simulink model "BATTERY_closed_loop"  (R2021a)
settings: Solver=VariableStepAuto  StartTime=0.0  StopTime=10  RelTol=1e-3
undefined symbols (not defined in the file): Ion, Lithium
libraries: spsSeriesRLCBranchLib x3, spsMosfetLib x2, spsBatteryLib x1, simulink x1, spsVoltageMeasurementLib x1, spspowerguiLib x1
settings Model: Creator=Bhargava  LastModifiedBy=Bhargava
settings SolverCC: ZeroCrossAlgorithm=Adaptive
settings DebuggingCC: MaskedZcDiagnostic=none  IgnoredZcDiagnostic=none

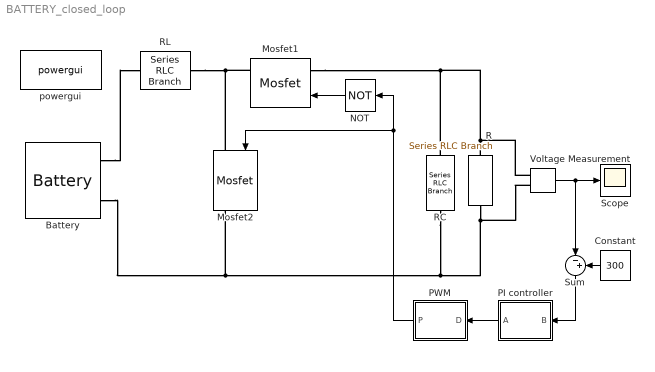
== system BATTERY_closed_loop ==
  " RC" : spsSeriesRLCBranchLib/Series RLC Branch  LConnTagsString=__new0  RConnTagsString=__new0  BranchType=RC  Resistance=0.1  Inductance=1e-3  SetiL0=off  InitialCurrent=0  Capacitance=520e-6  Setx0=off  InitialVoltage=0  Measurements=None
  Battery : spsBatteryLib/Battery  BatType=Lithium-Ion  ShowTempParam=off  ThermalPreset=no  ShowAgeParam=off  NomV=50  NomQ=15  SOC=100  Batt_Tr=30  PresetModel=off  MaxQ=15  MinV=37.5  FullV=120  Dis_rate=6.5217  R=0.033333  Normal_OP=13.5652  expZone="[54.0193     0.736957]"  current=[6.5 13 32.5]  Units=Time  Tci=20  NomT=20  T2=-30  MaxQ2=4.8  FullV2=7.1  Normal_OP2=5.655  expZone2="[6.58           1]"  Rca=0.6  ti=2000  Dp=0  Neq0=0  Tsim=1e6  Ta1=25  Qeol=5.4*0.9  Reol=0.013333*1.2  Char_age=[2.3478, 3]  Dis_age=[2.3478, 10]  N1=1500  N2=10500  N3=1000  N4=1400  Ta2=45  N5=950
  Constant : Constant  Value=300
  Mosfet1 : spsMosfetLib/Mosfet  Ron=0.1  Lon=0  Rd=0.01  Vfd=0  IC=0  Rs=1e5  Cs=inf  Measurements=on
  Mosfet2 : spsMosfetLib/Mosfet  Ron=0.1  Lon=0  Rd=0.01  Vfd=0  IC=0  Rs=1e5  Cs=inf  Measurements=on
  NOT : Logic  Operator=NOT  AllPortsSameDT=off  OutDataTypeStr=boolean
  PI controller : Subsystem
  PWM : Subsystem
  R : spsSeriesRLCBranchLib/Series RLC Branch  LConnTagsString=__new0  RConnTagsString=__new0  BranchType=R  Resistance=300  Inductance=353e-6  SetiL0=off  InitialCurrent=0  Capacitance=1e-6  Setx0=off  InitialVoltage=0  Measurements=None
  RL : spsSeriesRLCBranchLib/Series RLC Branch  LConnTagsString=__new0  RConnTagsString=__new0  BranchType=RL  Resistance=0.1  Inductance=353e-6  SetiL0=off  InitialCurrent=0  Capacitance=1e-6  Setx0=off  InitialVoltage=0  Measurements=None
  Scope : Scope
  Sum : Sum  Inputs=|-+
  Voltage Measurement : spsVoltageMeasurementLib/Voltage Measurement  PhasorSimulation=off  OutputType=Complex  PSBequivalent=0
  powergui : spspowerguiLib/powergui  Priority=1  SimulationMode=Discrete  SampleTime=20e-7  frequency=60  Iterations=50  frequencyindice=0  Pbase=100e6  ErrMax=1e-4  UnitsV=kV  UnitsW=MW  buscounter=0  FunctionMessages=off  echomessages=off  EnableUseOfTLC=off  CurrentSourceSwitches=off  DisableSnubberDevices=off  DisableRonSwitches=off  DisableVfSwitches=off  DisplayEquations=off  AutomaticDiscreteSolvers=off  SolverType=Tustin/Backward Euler (TBE)  Interpol=off  ExternalGateDelay=off  methode=off  Ts=100  x0status=blocks  SPID=on  SwTol=0  HookPort=off  NonlinearTolerance=1e-4  nMaxIteration=100  ContinueOnMaxIteration=off  RestoreLinks=warning  ResistiveCurrentMeasurement=off  Frange=[0:2:500]  Ylog=off  Xlog=on  ShowGrid=off  save=off  variable=ZData  structure=0  ZoomFFT=off  StartTime=0.0  cycles=1  DisplayStyle=1  fundamental=60  FreqAxis=off  MaxFrequency=1000  frequencyindicesteady=1  RmsSteady=1  display=off
  wires:
  Voltage Measurement/1 -> Scope/1, Sum/1
  NOT/1 -> Mosfet1/1
  Constant/1 -> Sum/2
  Sum/1 -> PI controller/1(B)
  PWM/1(P) -> NOT/1, Mosfet2/1
  PI controller/1(A) -> PWM/1(D)
  connections:
  Voltage Measurement/LConn2 -- Battery/LConn2 -- Mosfet2/RConn1 -- " RC"/RConn1 -- R/LConn1
  Battery/LConn1 -- RL/RConn1
  Voltage Measurement/LConn1 -- Mosfet1/LConn1 -- " RC"/LConn1 -- R/RConn1
  RL/LConn1 -- Mosfet1/RConn1 -- Mosfet2/LConn1

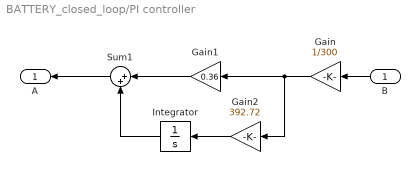
== system BATTERY_closed_loop/PI controller ==
  B : Inport
  Gain : Gain  Gain=1/300
  Gain1 : Gain  Gain=0.36
  Gain2 : Gain  Gain=392.72
  Integrator : Integrator
  Sum1 : Sum  Inputs=|++
  A : Outport
  wires:
  Gain2/1 -> Integrator/1
  B/1 -> Gain/1
  Gain1/1 -> Sum1/1
  Sum1/1 -> A/1
  Gain/1 -> Gain2/1, Gain1/1
  Integrator/1 -> Sum1/2

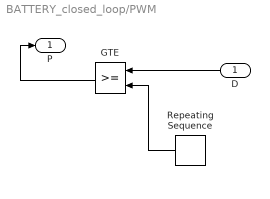
== system BATTERY_closed_loop/PWM ==
  D : Inport
  GTE : RelationalOperator  OutDataTypeStr=boolean  RndMeth=Simplest
  Repeating Sequence : simulink/Sources/Repeating Sequence  rep_seq_t=[0 1/20000]  rep_seq_y=[0 1]
  P : Outport
  wires:
  GTE/1 -> P/1
  Repeating Sequence/1 -> GTE/2
  D/1 -> GTE/1
